simulink model "ARPOD_Passive"  (R2019b)
settings: Solver=VariableStepAuto  StartTime=0.0  StopTime=240  RelTol=1e-3
model workspace (MAT data in the model file):
  x0_mode2 = Simulink.Parameter
  x0_mode2.DataType = 'auto'
  x0_mode2.Dimensions = [0 0]
values from neighbouring files (symbols this model uses):
  G11 = 3*n^2 -Glqr(1,1)/m    [init.m]
  G12 = -Glqr(1,2)/m    [init.m]
  G13 = -Glqr(1,3)/m    [init.m]
  G14 = 2*n -Glqr(1,4)/m    [init.m]
  G21 = -Glqr(2,1)/m    [init.m]
  G22 = -Glqr(2,2)/m    [init.m]
  G23 = -2*n -Glqr(2,3)/m    [init.m]
  G24 = -Glqr(2,4)/m    [init.m]
  J11 = 3*n^2 -Jlqr(1,1)/m    [init.m]
  J12 = -Jlqr(1,2)/m    [init.m]
  J13 = -Jlqr(1,3)/m    [init.m]
  J14 = 2*n -Jlqr(1,4)/m    [init.m]
  J21 = -Jlqr(2,1)/m    [init.m]
  J22 = -Jlqr(2,2)/m    [init.m]
  J23 = -2*n -Jlqr(2,3)/m    [init.m]
  J24 = -Jlqr(2,4)/m    [init.m]
  K11 = 3*n^2 -Klqr(1,1)/m    [init.m]
  K12 = -Klqr(1,2)/m    [init.m]
  K13 = -Klqr(1,3)/m    [init.m]
  K14 = 2*n -Klqr(1,4)/m    [init.m]
  K21 = -Klqr(2,1)/m    [init.m]
  K22 = -Klqr(2,2)/m    [init.m]
  K23 = -2*n -Klqr(2,3)/m    [init.m]
  K24 = -Klqr(2,4)/m    [init.m]
undefined symbols (not defined in the file or in its folder): vx0, vx0_mode2, vy0, vy0_mode2, x0, y0, y0_mode2
libraries: simulink x3
settings Model: Creator=yuxia  LastModifiedBy=yuxia

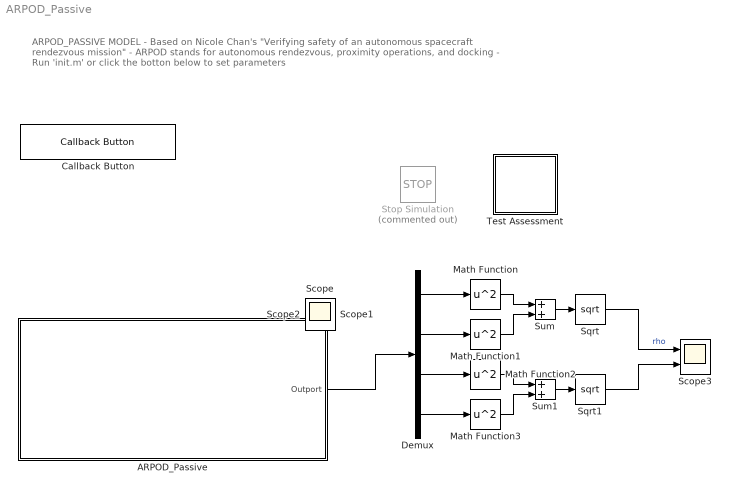
== system ARPOD_Passive ==
  note: ARPOD_PASSIVE MODEL
      |
      | - Based on Nicole Chan's "Verifying safety of an autonomous spacecraft rendezvous mission"
      | - ARPOD stands for autonomous rendezvous, proximity operations, and docking
      | - Run 'init.m' or click the botton below to set parameters
  ARPOD_Passive : Subsystem
  Callback Button : CallbackButton  ButtonText=CLICK TO INITIALIZE
      settings: ClickFcn=run 'init.m';
  Demux : Demux
  Math Function{,1..3} (4 alike) : Math  Operator=square  SignedPower=off  SaturateOnIntegerOverflow=on
  Scope3 : Scope  NumInputPorts=2
  Sqrt : Sqrt  SaturateOnIntegerOverflow=on
  Sqrt1 : Sqrt  SaturateOnIntegerOverflow=on
  Stop Simulation : Stop  Commented=on
  Sum : Sum
  Sum1 : Sum
  Test Assessment : Test Sequence  TreatAsAtomicUnit=on
  Scope : Scope
  Scope1 : Scope
  Scope2 : Scope
  wires:
  ARPOD_Passive/1(Outport) -> Demux/1
  Demux/1 -> Math Function/1
  Demux/2 -> Math Function1/1
  Math Function/1 -> Sum/1
  Math Function1/1 -> Sum/2
  Sum/1 -> Sqrt/1
  Sqrt/1 -> Scope3/1  "rho"
  Sum1/1 -> Sqrt1/1
  Math Function2/1 -> Sum1/1
  Math Function3/1 -> Sum1/2
  Demux/4 -> Math Function3/1
  Sqrt1/1 -> Scope3/2
  Demux/3 -> Math Function2/1

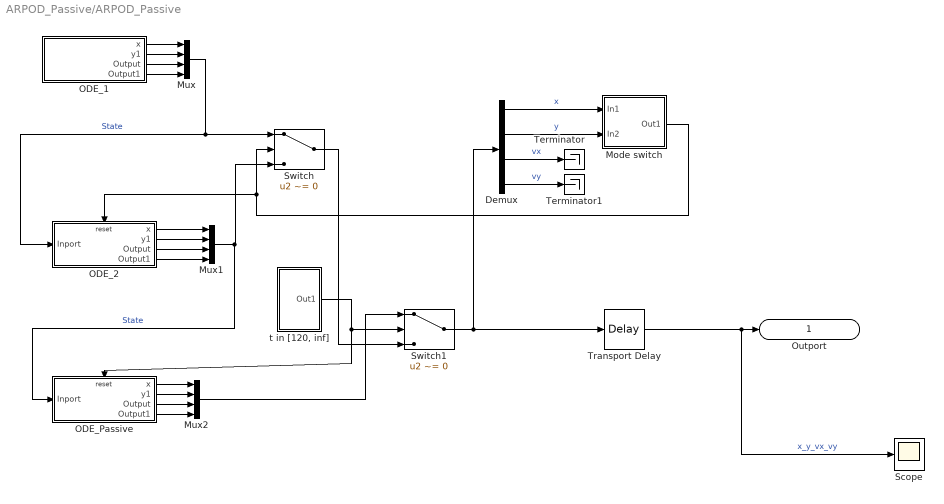
== system ARPOD_Passive/ARPOD_Passive ==
  Demux : Demux
  Mode switch : Subsystem
  Mux : Mux
  Mux1 : Mux
  Mux2 : Mux
  ODE_1 : Subsystem
  ODE_2 : Subsystem
  ODE_Passive : Subsystem
  Scope : Scope
  Switch : Switch  Criteria=u2 ~= 0  Threshold=1
  Switch1 : Switch  Criteria=u2 ~= 0  Threshold=1
  Terminator : Terminator
  Terminator1 : Terminator
  Transport Delay : TransportDelay  DelayTime=1e-6
  "t in [120, inf]" : Subsystem
  Outport : Outport
  wires:
  Demux/2 -> Mode switch/2(In2)  "y"
  "t in [120, inf]"/1(Out1) -> ODE_Passive/Reset, Switch1/2
  Mux1/1 -> ODE_Passive/1(Inport), Switch/3  "State"
  Mode switch/1(Out1) -> Switch/2, ODE_2/Reset
  ODE_2/4(Output1) -> Mux1/4
  ODE_Passive/2(y1) -> Mux2/2
  ODE_Passive/3(Output) -> Mux2/3
  Mux2/1 -> Switch1/1
  ODE_1/3(Output) -> Mux/3
  Switch/1 -> Switch1/3
  ODE_2/1(x) -> Mux1/1
  ODE_2/3(Output) -> Mux1/3
  Mux/1 -> Switch/1, ODE_2/1(Inport)  "State"
  ODE_Passive/4(Output1) -> Mux2/4
  Switch1/1 -> Transport Delay/1, Demux/1
  ODE_1/1(x) -> Mux/1
  Demux/3 -> Terminator/1  "vx"
  ODE_Passive/1(x) -> Mux2/1
  Demux/4 -> Terminator1/1  "vy"
  ODE_1/2(y1) -> Mux/2
  Demux/1 -> Mode switch/1(In1)  "x"
  ODE_2/2(y1) -> Mux1/2
  ODE_1/4(Output1) -> Mux/4
  Transport Delay/1 -> Scope/1, Outport/1  "x_y_vx_vy"

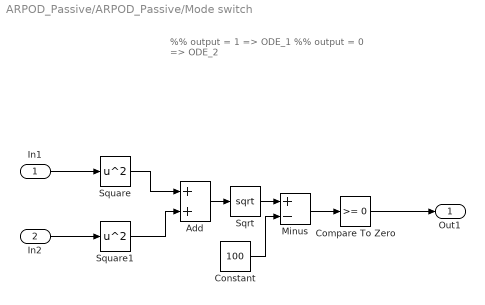
== system ARPOD_Passive/ARPOD_Passive/Mode switch ==
  note: %% output = 1 => ODE_1
      | %% output = 0 => ODE_2
  In1 : Inport
  In2 : Inport  Port=2
  Add : Sum
  Compare To Zero : simulink/Logic and Bit Operations/Compare To Zero  relop=>=  OutDataTypeStr=boolean
  Constant : Constant  Value=100
  Minus : Sum  Inputs=+-
  Sqrt : Sqrt  SaturateOnIntegerOverflow=on
  Square : Math  Operator=square  SignedPower=off  SaturateOnIntegerOverflow=on
  Square1 : Math  Operator=square  SignedPower=off  SaturateOnIntegerOverflow=on
  Out1 : Outport
  wires:
  Square/1 -> Add/1
  Square1/1 -> Add/2
  Constant/1 -> Minus/2
  Minus/1 -> Compare To Zero/1
  Compare To Zero/1 -> Out1/1
  Sqrt/1 -> Minus/1
  Add/1 -> Sqrt/1
  In1/1 -> Square/1
  In2/1 -> Square1/1

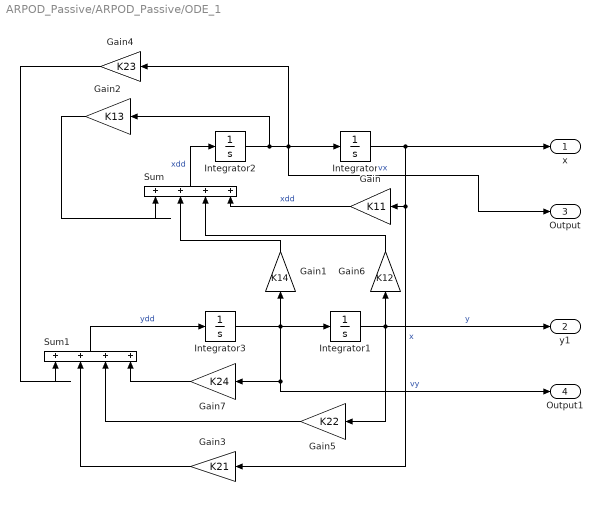
== system ARPOD_Passive/ARPOD_Passive/ODE_1 ==
  Gain : Gain  Gain=K11
  Gain1 : Gain  Gain=K14
  Gain2 : Gain  Gain=K13
  Gain3 : Gain  Gain=K21
  Gain4 : Gain  Gain=K23
  Gain5 : Gain  Gain=K22
  Gain6 : Gain  Gain=K12
  Gain7 : Gain  Gain=K24
  Integrator : Integrator  InitialCondition=x0
  Integrator1 : Integrator  InitialCondition=y0
  Integrator2 : Integrator  InitialCondition=vx0
  Integrator3 : Integrator  InitialCondition=vy0
  Sum : Sum  Inputs=|++++
  Sum1 : Sum  Inputs=|++++
  x : Outport
  y1 : Outport  Port=2
  Output : Outport  Port=3
  Output1 : Outport  Port=4
  wires:
  Gain1/1 -> Sum/2
  Gain5/1 -> Sum1/3
  Gain2/1 -> Sum/1
  Sum1/1 -> Integrator3/1  "ydd"
  Gain7/1 -> Sum1/4
  Gain3/1 -> Sum1/2
  Gain6/1 -> Sum/3
  Gain4/1 -> Sum1/1
  Integrator1/1 -> y1/1, Gain5/1, Gain6/1  "y"
  Integrator/1 -> x/1, Gain3/1, Gain/1  "x"
  Integrator2/1 -> Output/1, Gain4/1, Integrator/1, Gain2/1  "vx"
  Integrator3/1 -> Output1/1, Gain7/1, Integrator1/1, Gain1/1  "vy"
  Gain/1 -> Sum/4  "xdd"
  Sum/1 -> Integrator2/1  "xdd"

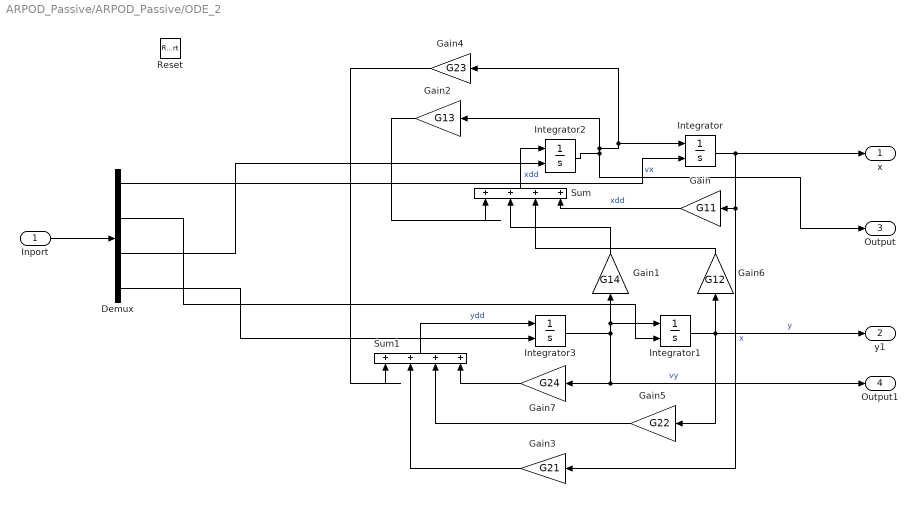
== system ARPOD_Passive/ARPOD_Passive/ODE_2 ==
  Inport : Inport
  Reset : ResetPort  DisableCoverage=on
  Demux : Demux
  Gain : Gain  Gain=G11
  Gain1 : Gain  Gain=G14
  Gain2 : Gain  Gain=G13
  Gain3 : Gain  Gain=G21
  Gain4 : Gain  Gain=G23
  Gain5 : Gain  Gain=G22
  Gain6 : Gain  Gain=G12
  Gain7 : Gain  Gain=G24
  Integrator : Integrator  InitialConditionSource=external  InitialCondition=x0_mode2
  Integrator1 : Integrator  InitialConditionSource=external  InitialCondition=y0_mode2
  Integrator2 : Integrator  InitialConditionSource=external  InitialCondition=vx0_mode2
  Integrator3 : Integrator  InitialConditionSource=external  InitialCondition=vy0_mode2
  Sum : Sum  Inputs=|++++
  Sum1 : Sum  Inputs=|++++
  x : Outport
  y1 : Outport  Port=2
  Output : Outport  Port=3
  Output1 : Outport  Port=4
  wires:
  Gain6/1 -> Sum/3
  Gain2/1 -> Sum/1
  Gain5/1 -> Sum1/3
  Gain/1 -> Sum/4  "xdd"
  Gain7/1 -> Sum1/4
  Gain3/1 -> Sum1/2
  Gain4/1 -> Sum1/1
  Sum/1 -> Integrator2/1  "xdd"
  Integrator/1 -> x/1, Gain3/1, Gain/1  "x"
  Sum1/1 -> Integrator3/1  "ydd"
  Integrator2/1 -> Gain4/1, Integrator/1, Gain2/1, Output/1  "vx"
  Integrator3/1 -> Integrator1/1, Gain1/1, Output1/1, Gain7/1  "vy"
  Gain1/1 -> Sum/2
  Integrator1/1 -> Gain6/1, y1/1, Gain5/1  "y"
  Inport/1 -> Demux/1
  Demux/1 -> Integrator/2
  Demux/2 -> Integrator1/2
  Demux/3 -> Integrator2/2
  Demux/4 -> Integrator3/2

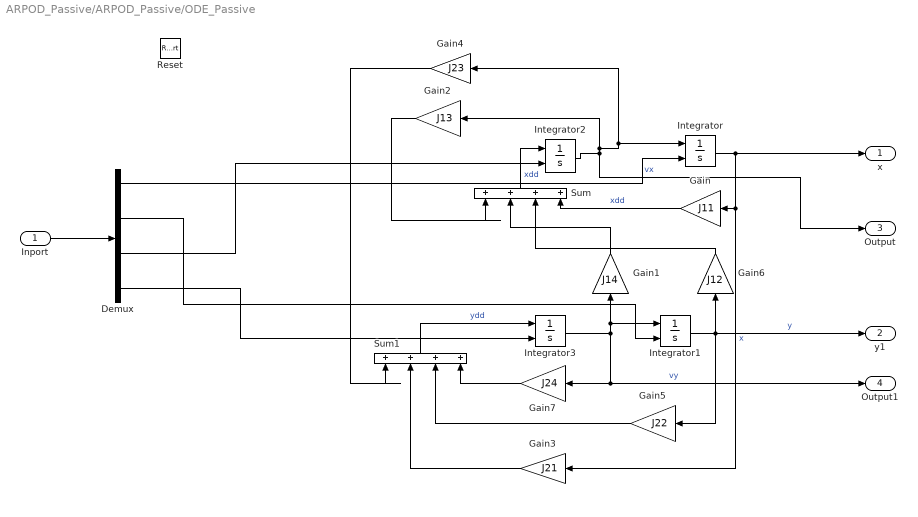
== system ARPOD_Passive/ARPOD_Passive/ODE_Passive ==
  Inport : Inport
  Reset : ResetPort  DisableCoverage=on
  Demux : Demux
  Gain : Gain  Gain=J11
  Gain1 : Gain  Gain=J14
  Gain2 : Gain  Gain=J13
  Gain3 : Gain  Gain=J21
  Gain4 : Gain  Gain=J23
  Gain5 : Gain  Gain=J22
  Gain6 : Gain  Gain=J12
  Gain7 : Gain  Gain=J24
  Integrator : Integrator  InitialConditionSource=external  InitialCondition=x0_mode2
  Integrator1 : Integrator  InitialConditionSource=external  InitialCondition=y0_mode2
  Integrator2 : Integrator  InitialConditionSource=external  InitialCondition=vx0_mode2
  Integrator3 : Integrator  InitialConditionSource=external  InitialCondition=vy0_mode2
  Sum : Sum  Inputs=|++++
  Sum1 : Sum  Inputs=|++++
  x : Outport
  y1 : Outport  Port=2
  Output : Outport  Port=3
  Output1 : Outport  Port=4
  wires:
  Gain6/1 -> Sum/3
  Gain2/1 -> Sum/1
  Gain5/1 -> Sum1/3
  Gain/1 -> Sum/4  "xdd"
  Gain7/1 -> Sum1/4
  Gain3/1 -> Sum1/2
  Gain4/1 -> Sum1/1
  Sum/1 -> Integrator2/1  "xdd"
  Integrator/1 -> x/1, Gain3/1, Gain/1  "x"
  Sum1/1 -> Integrator3/1  "ydd"
  Integrator2/1 -> Gain4/1, Integrator/1, Gain2/1, Output/1  "vx"
  Integrator3/1 -> Integrator1/1, Gain1/1, Output1/1, Gain7/1  "vy"
  Gain1/1 -> Sum/2
  Integrator1/1 -> Gain6/1, y1/1, Gain5/1  "y"
  Inport/1 -> Demux/1
  Demux/1 -> Integrator/2
  Demux/2 -> Integrator1/2
  Demux/3 -> Integrator2/2
  Demux/4 -> Integrator3/2

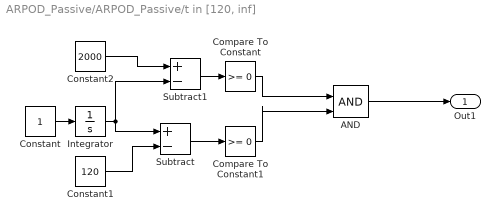
== system ARPOD_Passive/ARPOD_Passive/t in [120, inf] ==
  AND : Logic  IconShape=distinctive  AllPortsSameDT=off  OutDataTypeStr=boolean
  Compare To Constant : simulink/Logic and Bit Operations/Compare To Constant  relop=>=  const=0  OutDataTypeStr=boolean
  Compare To Constant1 : simulink/Logic and Bit Operations/Compare To Constant  relop=>=  const=0  OutDataTypeStr=boolean
  Constant : Constant
  Constant1 : Constant  Value=120
  Constant2 : Constant  Value=2000
  Integrator : Integrator
  Subtract : Sum  Inputs=+-
  Subtract1 : Sum  Inputs=+-
  Out1 : Outport
  wires:
  Constant1/1 -> Subtract/2
  Subtract/1 -> Compare To Constant1/1
  AND/1 -> Out1/1
  Integrator/1 -> Subtract1/2, Subtract/1
  Constant/1 -> Integrator/1
  Constant2/1 -> Subtract1/1
  Subtract1/1 -> Compare To Constant/1
  Compare To Constant/1 -> AND/1
  Compare To Constant1/1 -> AND/2

== stateflow chart ARPOD_Passive/Test Assessment ==
  settings: stateMachineType=SIMPLIFIED_MACHINE
  state step_1
    state step_1_1
    state step_1_2
    (default) -> (junction 22)
    step_1 -> (junction 22)
    (junction 22) -> (junction 23) [order 1] : [t < 5]
    (junction 23) -> step_1_1 [order 1] : [~in(step_1_1)]
    (junction 23) -> (junction 26) [order 2]
    (junction 31) -> (junction 32)
    (junction 32) -> step_1_2 [order 1] : [~in(step_1_2)]
    (junction 32) -> (junction 35) [order 2]
    (junction 22) -> (junction 31) [order 2]
  (default) -> step_1
